simulink model "Hw03_P3"  (R2024a)
settings: Solver=VariableStepAuto  StartTime=0.0  StopTime=10.0  RelTol=1e-3
InitFcn:
  | if ~ evalin('base', 'exist(''C1_Hinf'', ''var'')')
  |     C1_Hinf = load('C1_hinf').C1;
  | end
  | 
  | if ~ evalin('base', 'exist(''C2_Hinf'', ''var'')')
  |     C2_Hinf = load('C2_hinf').C2;
  | end
  | 
  | if ~ evalin('base', 'exist(''C_Musyn'', ''var'')')
  |     C_Musyn = load('C_musyn.mat').C_mu;
  | end
undefined symbols (not defined in the file or in its folder): minreal
libraries: cstblocks x3, simulink x2
settings Model: Creator=bojack  LastModifiedBy=bojack

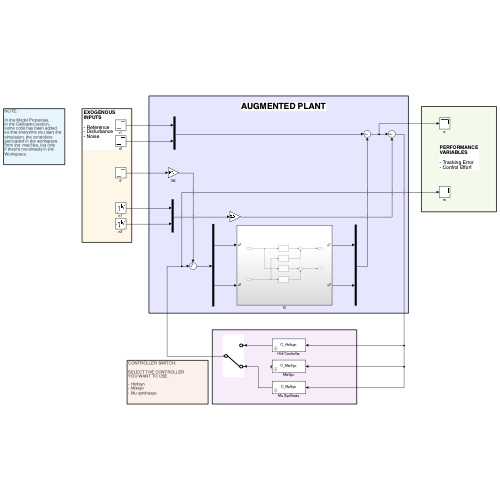
[thumbnail: Simulink's stored preview of the top-level diagram]
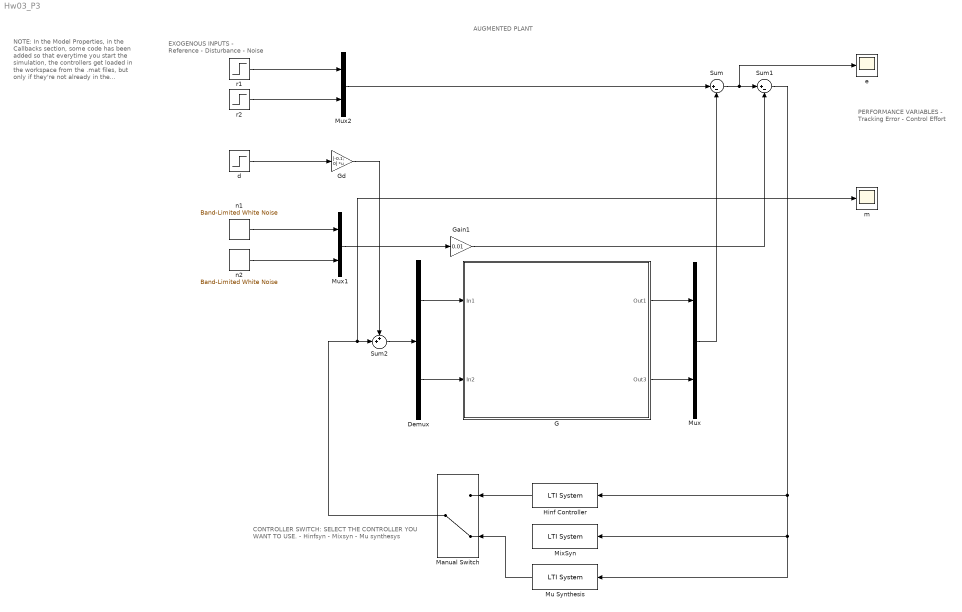
== system Hw03_P3 ==
  note: NOTE:
      |
      | In the Model Properties,
      | in the Callbacks section,
      | some code has been added
      | so that everytime you start the
      | simulation, the controllers
      | get loaded in the workspace
      | from the .mat files, but only
      | if they're not already in the
      | Workspace.
  note: CONTROLLER SWITCH:
      |
      | SELECT THE CONTROLLER
      | YOU WANT TO USE.
      |
      | - Hinfsyn
      | - Mixsyn
      | - Mu synthesys
  note: AUGMENTED PLANT
  note: PERFORMANCE
      | VARIABLES
      |
      | - Tracking Error
      | - Control Effort
  note: EXOGENOUS
      | INPUTS
      |
      | - Reference
      | - Disturbance
      | - Noise
  Demux : Demux  Outputs=2
  G : Subsystem
  Gain1 : Gain  Gain=0.01
  Gd : Gain  Gain=[-0.1; 0]  Multiplication=Matrix(K*u)
  Hinf Controller : cstblocks/LTI System  sys=tf(minreal(C1_Hinf))  IC=[]  PadeOrder=0  mask(LTI Block){}
      mask Display: disp("C_Hinfsyn")
  Manual Switch : ManualSwitch  CurrentSetting=0
  MixSyn : cstblocks/LTI System  sys=tf(minreal(C2_Hinf))  IC=[]  PadeOrder=0  mask(LTI Block){}
      mask Display: disp('C_MixSyn')
  Mu Synthesis : cstblocks/LTI System  sys=C_Musyn  IC=[]  PadeOrder=0  mask(LTI Block){}
      mask Display: disp('C_MuSyn')
  Mux : Mux  Inputs=2
  Mux1 : Mux  Inputs=2
  Mux2 : Mux  Inputs=2
  Sum : Sum  Inputs=|+-
  Sum1 : Sum  Inputs=|+-
  Sum2 : Sum  Inputs=++|
  d : Step  Time=0  After=0.1  SampleTime=0
  e : Scope
  m : Scope
  n1 : simulink/Sources/Band-Limited White Noise  Cov=[0.01]  Ts=0.1  seed=[23341]
  n2 : simulink/Sources/Band-Limited White Noise  Cov=[0.01]  Ts=0.1  seed=[23341]
  r1 : Step  Time=0  After=0.5  SampleTime=0
  r2 : Step  Time=0  After=1.5  SampleTime=0
  wires:
  G/1(Out1) -> Mux/1
  G/2(Out3) -> Mux/2
  Demux/1 -> G/1(In1)
  Demux/2 -> G/2(In2)
  Sum/1 -> e/1, Sum1/1
  d/1 -> Gd/1
  n1/1 -> Mux1/1
  n2/1 -> Mux1/2
  Mux1/1 -> Gain1/1
  Mux/1 -> Sum/2
  Sum2/1 -> Demux/1
  Gd/1 -> Sum2/1
  Gain1/1 -> Sum1/2
  r2/1 -> Mux2/2
  r1/1 -> Mux2/1
  Mux2/1 -> Sum/1
  Hinf Controller/1 -> Manual Switch/1
  Manual Switch/1 -> Sum2/2, m/1
  Sum1/1 -> Hinf Controller/1, MixSyn/1, Mu Synthesis/1
  Mu Synthesis/1 -> Manual Switch/2

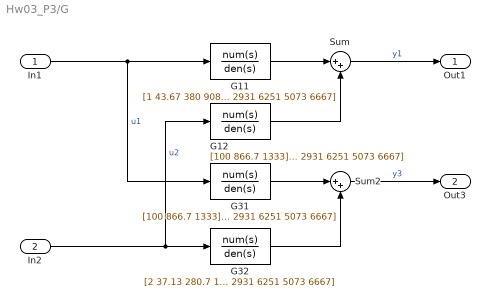
== system Hw03_P3/G ==
  In1 : Inport
  In2 : Inport  Port=2
  G11 : TransferFcn  Numerator=[1 43.67 380 908 1333]  Denominator=[1 48.77 601.1 2931 6251 5073 6667]
  G12 : TransferFcn  Numerator=[100 866.7 1333]  Denominator=[1 48.77 601.1 2931 6251 5073 6667]
  G31 : TransferFcn  Numerator=[100 866.7 1333]  Denominator=[1 48.77 601.1 2931 6251 5073 6667]
  G32 : TransferFcn  Numerator=[2 37.13 280.7 1019 2067]  Denominator=[1 48.77 601.1 2931 6251 5073 6667]
  Sum : Sum  Inputs=|++
  Sum2 : Sum  Inputs=|++
  Out1 : Outport
  Out3 : Outport  Port=2
  wires:
  Sum2/1 -> Out3/1  "y3"
  G32/1 -> Sum2/2
  In2/1 -> G32/1, G12/1  "u2"
  G12/1 -> Sum/2
  G11/1 -> Sum/1
  G31/1 -> Sum2/1
  In1/1 -> G11/1, G31/1  "u1"
  Sum/1 -> Out1/1  "y1"
